simulink model "R_estimation"  (R2021a)
settings: Solver=ode3  StartTime=0.0  StopTime=60  FixedStep=t_sim  RelTol=1e-3
values from neighbouring files (symbols this model uses):
  eul_0 = [0;0;0]    [Q_parameter.m]    (also in R_parameter.m)
  ki = 0.3    [R_parameter.m]
  kp = 1    [R_parameter.m]
  Q0 = G0*G0'    [R_parameter.m]
  t_h = 4e-2    (= 0.04)    [Q_parameter.m]    (also in R_parameter.m)
  t_sim = 1e-3    (= 0.001)    [Q_parameter.m]    (also in R_parameter.m)
undefined symbols (not defined in the file or in its folder): DiscIntNeverNeededParam
libraries: sharedtransform x3, sharedutil x2, shared6dofsys x1
settings Model: Creator=quangtruc  LastModifiedBy=quangtruc

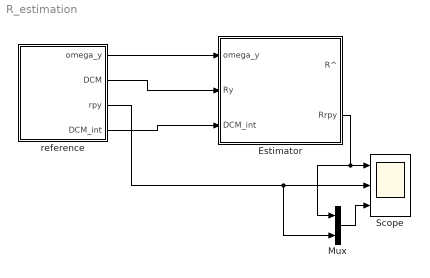
== system R_estimation ==
  Estimator : Subsystem
  Mux : Mux  Inputs=2
  Scope : Scope  NumInputPorts=3
  reference : Subsystem
  wires:
  reference/1(omega_y) -> Estimator/1(omega_y)
  reference/2(DCM) -> Estimator/2(Ry)
  reference/4(DCM_int) -> Estimator/3(DCM_int)
  Estimator/2(Rrpy) -> Mux/1, Scope/1
  reference/3(rpy) -> Mux/2, Scope/2
  Mux/1 -> Scope/3

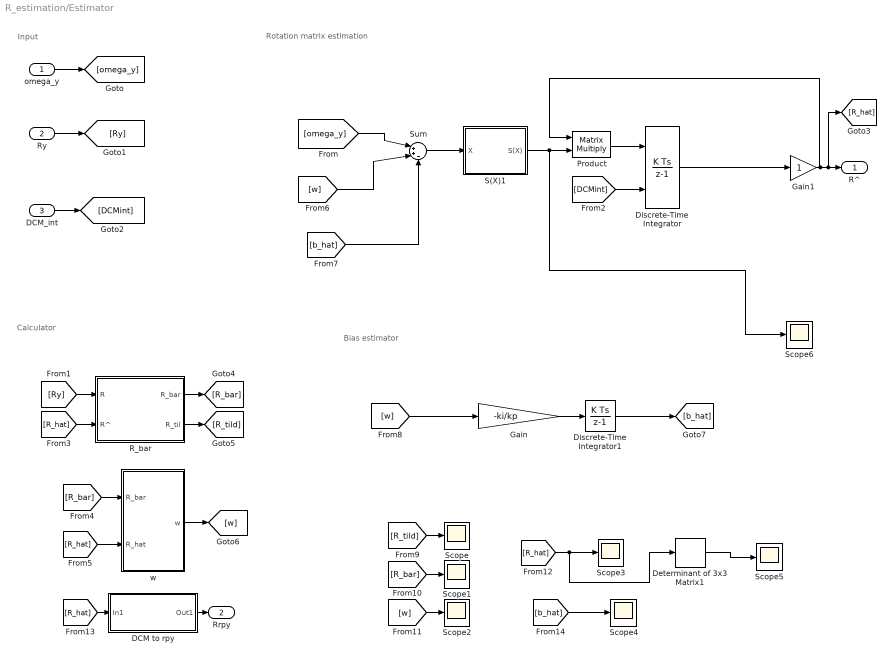
== system R_estimation/Estimator ==
  note: Bias estimator
  note: Calculator
  note: Input
  note: Rotation matrix estimation
  omega_y : Inport
  Ry : Inport  Port=2
  DCM_int : Inport  Port=3
  DCM to rpy : Subsystem
  Determinant of 3x3 Matrix1 : sharedutil/Determinant of 3x3 Matrix  aMode=aMode
      settings: SourceProductBaseCode=AE,PW,DR,MT,UV,VE
  Discrete-Time Integrator : DiscreteIntegrator  InitialConditionSource=external  SampleTime=t_sim  ICPrevOutput=DiscIntNeverNeededParam  ICPrevScaledInput=DiscIntNeverNeededParam
  Discrete-Time Integrator1 : DiscreteIntegrator  SampleTime=t_sim  ICPrevOutput=DiscIntNeverNeededParam  ICPrevScaledInput=DiscIntNeverNeededParam
  Gain : Gain  Gain=-ki/kp
  Gain1 : Gain
  Product : Product  Multiplication=Matrix(*)
  R_bar : Subsystem
  S(X)1 : Subsystem
  Scope{,1..6} (7 alike) : Scope
  Sum : Sum  Inputs=|++-
  w : Subsystem
  R^ : Outport
  Rrpy : Outport  Port=2
  wires:
  omega_y/1 -> [omega_y]
  Ry/1 -> [Ry]
  DCM_int/1 -> [DCMint]
  [R_hat] -> R_bar/2(R^)
  [Ry] -> R_bar/1(R)
  R_bar/1(R_bar) -> [R_bar]
  R_bar/2(R_til) -> [R_tild]
  [R_bar] -> w/1(R_bar)
  [R_hat] -> w/2(R_hat)
  S(X)1/1(S(X)) -> Scope6/1, Product/2
  [DCMint] -> Discrete-Time Integrator/2
  Sum/1 -> S(X)1/1(X)
  w/1(w) -> [w]
  [omega_y] -> Sum/1
  [w] -> Sum/2
  [b_hat] -> Sum/3
  [w] -> Gain/1
  Gain/1 -> Discrete-Time Integrator1/1
  Discrete-Time Integrator1/1 -> [b_hat]
  [R_tild] -> Scope/1
  [R_bar] -> Scope1/1
  [w] -> Scope2/1
  [R_hat] -> Determinant of 3x3 Matrix1/1, Scope3/1
  Discrete-Time Integrator/1 -> Gain1/1
  Gain1/1 -> Product/1, [R_hat], R^/1
  Product/1 -> Discrete-Time Integrator/1
  [R_hat] -> DCM to rpy/1(In1)
  DCM to rpy/1(Out1) -> Rrpy/1
  [b_hat] -> Scope4/1
  Determinant of 3x3 Matrix1/1 -> Scope5/1

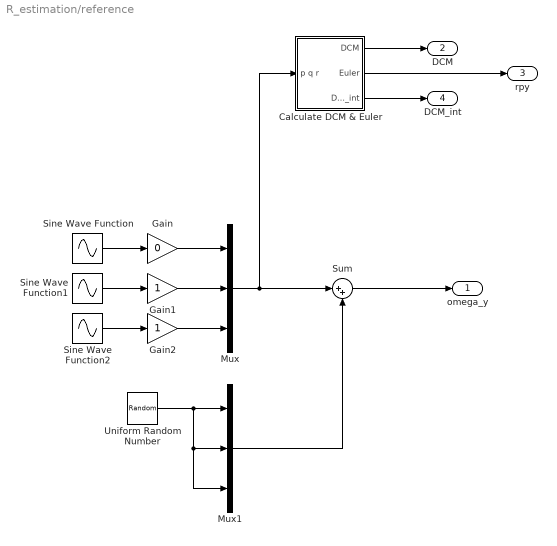
== system R_estimation/reference ==
  "Calculate DCM & Euler " : Subsystem
  Gain : Gain  Gain=0
  Gain1 : Gain
  Gain2 : Gain
  Mux : Mux  Inputs=3
  Mux1 : Mux  Inputs=3
  Sine Wave Function : Sin  SampleTime=0
  Sine Wave Function1 : Sin  Amplitude=0.1  Frequency=0.01  SampleTime=0
  Sine Wave Function2 : Sin  Amplitude=0.5  Frequency=0.5  SampleTime=0
  Sum : Sum  Inputs=|++
  Uniform Random Number : UniformRandomNumber  Minimum=-0.05  Maximum=0.05  SampleTime=t_h
  omega_y : Outport
  DCM : Outport  Port=2
  rpy : Outport  Port=3
  DCM_int : Outport  Port=4
  wires:
  "Calculate DCM & Euler "/1(DCM) -> DCM/1
  "Calculate DCM & Euler "/3(DCM_int) -> DCM_int/1
  "Calculate DCM & Euler "/2(Euler) -> rpy/1
  Gain/1 -> Mux/1
  Sine Wave Function/1 -> Gain/1
  Sine Wave Function1/1 -> Gain1/1
  Sine Wave Function2/1 -> Gain2/1
  Gain1/1 -> Mux/2
  Gain2/1 -> Mux/3
  Mux/1 -> "Calculate DCM & Euler "/1("p q r "), Sum/1
  Uniform Random Number/1 -> Mux1/3, Mux1/2, Mux1/1
  Mux1/1 -> Sum/2
  Sum/1 -> omega_y/1

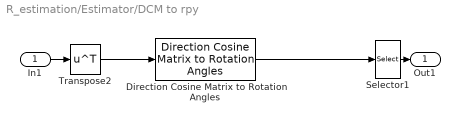
== system R_estimation/Estimator/DCM to rpy ==
  In1 : Inport
  Direction Cosine Matrix to Rotation Angles : sharedtransform/Direction Cosine Matrix to Rotation Angles  rotationOrder=ZYX  aMode=aMode  action=None  tolerance=eps(2)
      settings: SourceProductBaseCode=AE,PW,DR,MT,UV,VE
  Selector1 : Selector  InputPortWidth=3  IndexOptions=Index vector (dialog)  Indices=[3 2 1]  OutputSizes=1
  Transpose2 : Math  Operator=transpose  SignedPower=on  SaturateOnIntegerOverflow=on
  Out1 : Outport
  wires:
  Direction Cosine Matrix to Rotation Angles/1 -> Selector1/1
  Selector1/1 -> Out1/1
  In1/1 -> Transpose2/1
  Transpose2/1 -> Direction Cosine Matrix to Rotation Angles/1

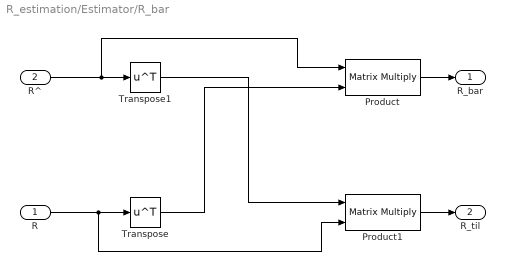
== system R_estimation/Estimator/R_bar ==
  R : Inport
  R^ : Inport  Port=2
  Product : Product  Multiplication=Matrix(*)
  Product1 : Product  Multiplication=Matrix(*)
  Transpose : Math  Operator=transpose  SignedPower=on  SaturateOnIntegerOverflow=on
  Transpose1 : Math  Operator=transpose  SignedPower=on  SaturateOnIntegerOverflow=on
  R_bar : Outport
  R_til : Outport  Port=2
  wires:
  Product/1 -> R_bar/1
  Product1/1 -> R_til/1
  Transpose1/1 -> Product1/1
  Transpose/1 -> Product/2
  R/1 -> Product1/2, Transpose/1
  R^/1 -> Product/1, Transpose1/1

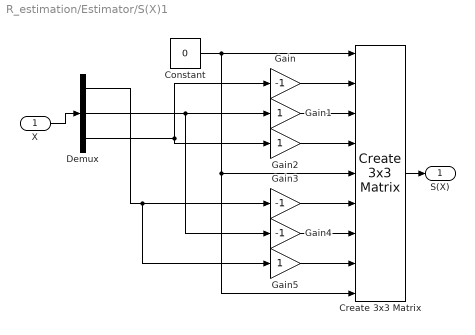
== system R_estimation/Estimator/S(X)1 ==
  X : Inport
  Constant : Constant  Value=0
  Create 3x3 Matrix : sharedutil/Create 3x3 Matrix  aMode=aMode
      settings: SourceProductBaseCode=AE,PW,DR,MT,UV,VE
  Demux : Demux  Outputs=3
  Gain : Gain  Gain=-1
  Gain1 : Gain
  Gain2 : Gain
  Gain3 : Gain  Gain=-1
  Gain4 : Gain  Gain=-1
  Gain5 : Gain
  S(X) : Outport
  wires:
  Create 3x3 Matrix/1 -> S(X)/1
  X/1 -> Demux/1
  Gain/1 -> Create 3x3 Matrix/2
  Constant/1 -> Create 3x3 Matrix/9, Create 3x3 Matrix/5, Create 3x3 Matrix/1
  Gain1/1 -> Create 3x3 Matrix/3
  Gain2/1 -> Create 3x3 Matrix/4
  Gain3/1 -> Create 3x3 Matrix/6
  Gain4/1 -> Create 3x3 Matrix/7
  Gain5/1 -> Create 3x3 Matrix/8
  Demux/3 -> Gain/1, Gain2/1
  Demux/2 -> Gain4/1, Gain1/1
  Demux/1 -> Gain5/1, Gain3/1

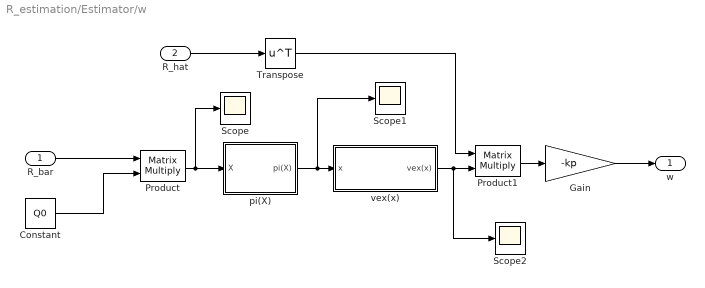
== system R_estimation/Estimator/w ==
  R_bar : Inport
  R_hat : Inport  Port=2
  Constant : Constant  Value=Q0
  Gain : Gain  Gain=-kp
  Product : Product  Multiplication=Matrix(*)
  Product1 : Product  Multiplication=Matrix(*)
  Scope : Scope
  Scope1 : Scope
  Scope2 : Scope
  Transpose : Math  Operator=transpose  SignedPower=on  SaturateOnIntegerOverflow=on
  pi(X) : Subsystem
  vex(x) : Subsystem
  w : Outport
  wires:
  R_bar/1 -> Product/1
  Constant/1 -> Product/2
  R_hat/1 -> Transpose/1
  Product/1 -> Scope/1, pi(X)/1(X)
  pi(X)/1(pi(X)) -> Scope1/1, vex(x)/1(x)
  vex(x)/1(vex(x)) -> Scope2/1, Product1/2
  Transpose/1 -> Product1/1
  Product1/1 -> Gain/1
  Gain/1 -> w/1

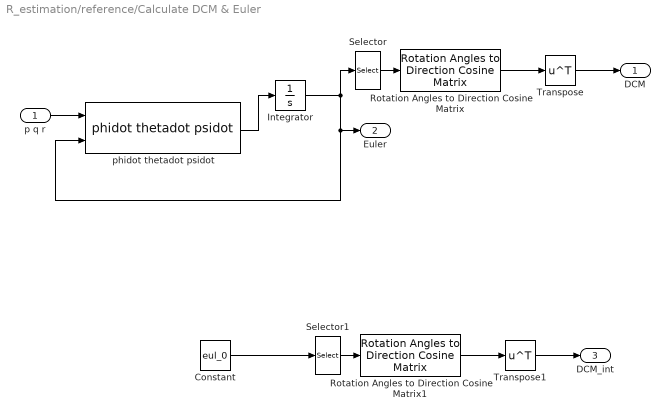
== system R_estimation/reference/Calculate DCM & Euler  ==
  "p q r " : Inport
  Constant : Constant  Value=eul_0
  Integrator : Integrator
  Rotation Angles to Direction Cosine Matrix : sharedtransform/Rotation Angles to Direction Cosine Matrix  rotationOrder=ZYX  aMode=aMode
      settings: SourceProductBaseCode=AE,PW,DR,MT,UV,VE
  Rotation Angles to Direction Cosine Matrix1 : sharedtransform/Rotation Angles to Direction Cosine Matrix  rotationOrder=ZYX  aMode=aMode
      settings: SourceProductBaseCode=AE,PW,DR,MT,UV,VE
  Selector : Selector  InputPortWidth=3  IndexOptions=Index vector (dialog)  Indices=[3 2 1]  OutputSizes=1
  Selector1 : Selector  InputPortWidth=3  IndexOptions=Index vector (dialog)  Indices=[3 2 1]  OutputSizes=1
  Transpose : Math  Operator=transpose  SignedPower=on  SaturateOnIntegerOverflow=on
  Transpose1 : Math  Operator=transpose  SignedPower=on  SaturateOnIntegerOverflow=on
  phidot thetadot psidot : shared6dofsys/DCM & Euler Angles (Euler)/phidot thetadot psidot  SystemSampleTime=-1  VariantActivationTime=update diagram  Latency=0  AutoFrameSizeCalculation=off
      settings: SourceProductBaseCode=AE,PW,DR,MT,UV,VE
  DCM : Outport  VectorParamsAs1DForOutWhenUnconnected=off
  Euler : Outport  Port=2  VectorParamsAs1DForOutWhenUnconnected=off
  DCM_int : Outport  Port=3  VectorParamsAs1DForOutWhenUnconnected=off
  wires:
  phidot thetadot psidot/1 -> Integrator/1
  "p q r "/1 -> phidot thetadot psidot/1
  Integrator/1 -> Euler/1, phidot thetadot psidot/2, Selector/1
  Selector/1 -> Rotation Angles to Direction Cosine Matrix/1
  Rotation Angles to Direction Cosine Matrix/1 -> Transpose/1
  Transpose/1 -> DCM/1
  Rotation Angles to Direction Cosine Matrix1/1 -> Transpose1/1
  Transpose1/1 -> DCM_int/1
  Selector1/1 -> Rotation Angles to Direction Cosine Matrix1/1
  Constant/1 -> Selector1/1

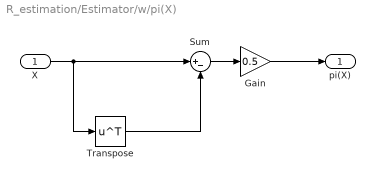
== system R_estimation/Estimator/w/pi(X) ==
  X : Inport
  Gain : Gain  Gain=0.5
  Sum : Sum  Inputs=|+-
  Transpose : Math  Operator=transpose  SignedPower=on  SaturateOnIntegerOverflow=on
  pi(X) : Outport
  wires:
  X/1 -> Sum/1, Transpose/1
  Transpose/1 -> Sum/2
  Sum/1 -> Gain/1
  Gain/1 -> pi(X)/1

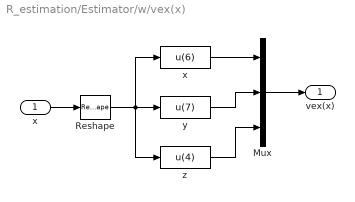
== system R_estimation/Estimator/w/vex(x) ==
  x : Inport
  Mux : Mux  Inputs=3
  Reshape : Reshape
  "x " : Fcn  Expr=u(6)
  y : Fcn  Expr=u(7)
  z : Fcn  Expr=u(4)
  vex(x) : Outport
  wires:
  x/1 -> Reshape/1
  "x "/1 -> Mux/1
  Reshape/1 -> z/1, y/1, "x "/1
  y/1 -> Mux/2
  z/1 -> Mux/3
  Mux/1 -> vex(x)/1
